simulink model "FDM_Degradation_oglm"  (R2020b)
settings: Solver=ode23tb  StartTime=0.0  StopTime=t_final  MaxStep=0.1  RelTol=1e-3
values from neighbouring files (symbols this model uses):
  initial_50_n = [0.015535 0.015535 0.015535 0.015535 0.015535 0.015535 0.015535 0.015535 0.015535 0.015535 0.015535 0.015535 ... (49 elements, 1x49)]    [LM_0.mat]    (also in RUn_Model_FDM.m = repmat(C_avg_n, 1, 49))
settings Model: Creator=moonjihoon  LastModifiedBy=moonjihoon

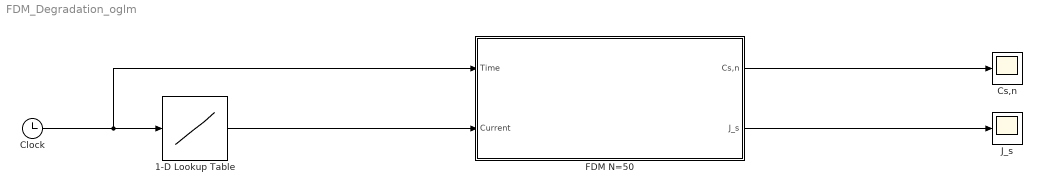
== system FDM_Degradation_oglm ==
  1-D Lookup Table : Lookup_n-D  NumberOfTableDimensions=1  BreakpointsForDimension1=t  Table=u  InternalRulePriority=Speed  RndMeth=Simplest  InputSameDT=on
  Clock : Clock
  Cs,n : Scope
  "FDM N=50 " : Subsystem
  J_s : Scope
  wires:
  1-D Lookup Table/1 -> "FDM N=50 "/2(Current)
  Clock/1 -> 1-D Lookup Table/1, "FDM N=50 "/1(Time)
  "FDM N=50 "/2(J_s) -> J_s/1
  "FDM N=50 "/1(Cs,n) -> Cs,n/1

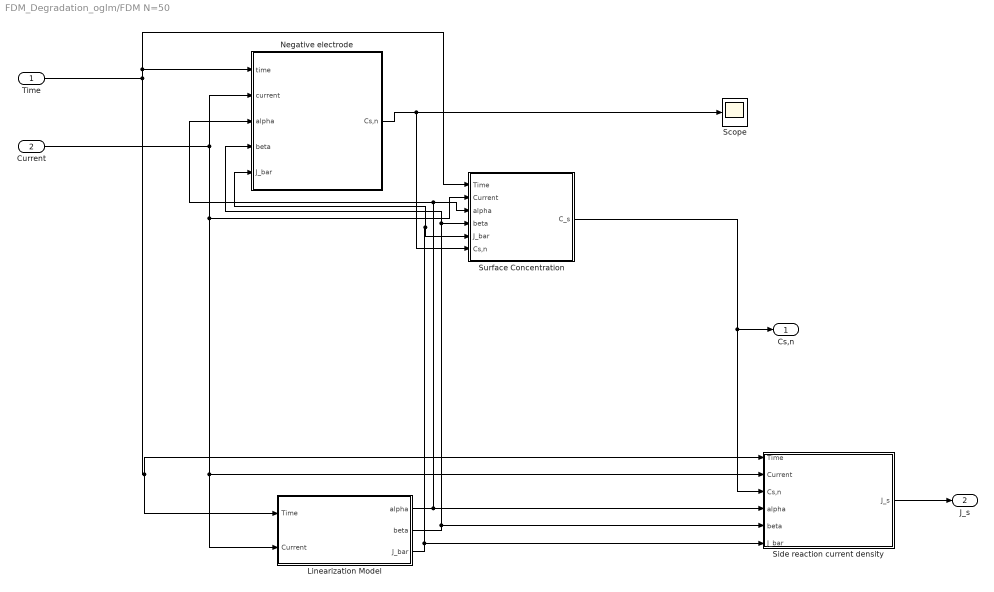
== system FDM_Degradation_oglm/FDM N=50  ==
  Time : Inport
  Current : Inport  Port=2
  Linearization Model : Subsystem
  Negative electrode : Subsystem
  Scope : Scope
  Side reaction current density : Subsystem
  Surface Concentration : Subsystem
  Cs,n : Outport
  J_s : Outport  Port=2
  wires:
  Negative electrode/1(Cs,n) -> Scope/1, Surface Concentration/6(Cs,n)
  Linearization Model/2(beta) -> Side reaction current density/5(beta), Negative electrode/4(beta), Surface Concentration/4(beta)
  Side reaction current density/1(J_s) -> J_s/1
  Linearization Model/1(alpha) -> Side reaction current density/4(alpha), Negative electrode/3(alpha), Surface Concentration/3(alpha)
  Time/1 -> Surface Concentration/1(Time), Negative electrode/1(time), Linearization Model/1(Time), Side reaction current density/1(Time)
  Surface Concentration/1(C_s) -> Side reaction current density/3(Cs,n), Cs,n/1
  Linearization Model/3(J_bar) -> Side reaction current density/6(J_bar), Negative electrode/5(J_bar), Surface Concentration/5(J_bar)
  Current/1 -> Surface Concentration/2(Current), Linearization Model/2(Current), Side reaction current density/2(Current), Negative electrode/2(current)

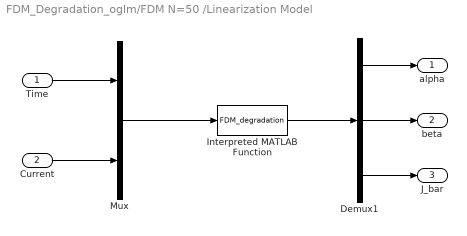
== system FDM_Degradation_oglm/FDM N=50 /Linearization Model ==
  Time : Inport
  Current : Inport  Port=2
  Demux1 : Demux  Outputs=3
  Interpreted MATLAB Function : MATLABFcn  MATLABFcn=FDM_degradation
  Mux : Mux  Inputs=2
  alpha : Outport
  beta : Outport  Port=2
  J_bar : Outport  Port=3
  wires:
  Demux1/1 -> alpha/1
  Demux1/3 -> J_bar/1
  Current/1 -> Mux/2
  Time/1 -> Mux/1
  Interpreted MATLAB Function/1 -> Demux1/1
  Demux1/2 -> beta/1
  Mux/1 -> Interpreted MATLAB Function/1

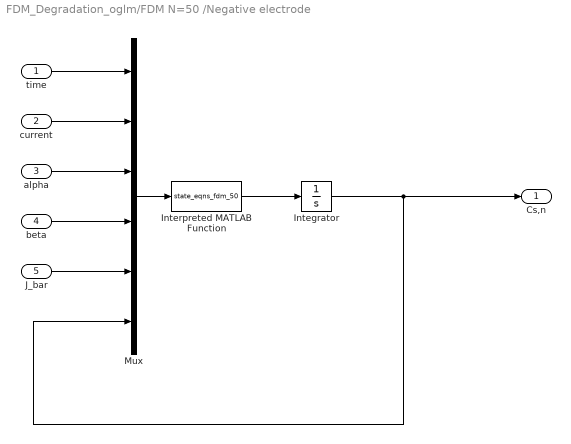
== system FDM_Degradation_oglm/FDM N=50 /Negative electrode ==
  time : Inport
  current : Inport  Port=2
  alpha : Inport  Port=3
  beta : Inport  Port=4
  J_bar : Inport  Port=5
  Integrator : Integrator  InitialCondition=initial_50_n
  Interpreted MATLAB Function : MATLABFcn  MATLABFcn=state_eqns_fdm_50
  Mux : Mux  Inputs=6
  Cs,n : Outport
  wires:
  Interpreted MATLAB Function/1 -> Integrator/1
  time/1 -> Mux/1
  current/1 -> Mux/2
  Mux/1 -> Interpreted MATLAB Function/1
  Integrator/1 -> Mux/6, Cs,n/1
  J_bar/1 -> Mux/5
  beta/1 -> Mux/4
  alpha/1 -> Mux/3

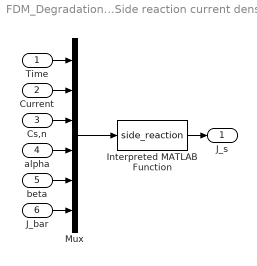
== system FDM_Degradation_oglm/FDM N=50 /Side reaction current density ==
  Time : Inport
  Current : Inport  Port=2
  Cs,n : Inport  Port=3
  alpha : Inport  Port=4
  beta : Inport  Port=5
  J_bar : Inport  Port=6
  Interpreted MATLAB Function : MATLABFcn  MATLABFcn=side_reaction
  Mux : Mux  Inputs=6
  J_s : Outport
  wires:
  Interpreted MATLAB Function/1 -> J_s/1
  Time/1 -> Mux/1
  Current/1 -> Mux/2
  Mux/1 -> Interpreted MATLAB Function/1
  J_bar/1 -> Mux/6
  beta/1 -> Mux/5
  alpha/1 -> Mux/4
  Cs,n/1 -> Mux/3

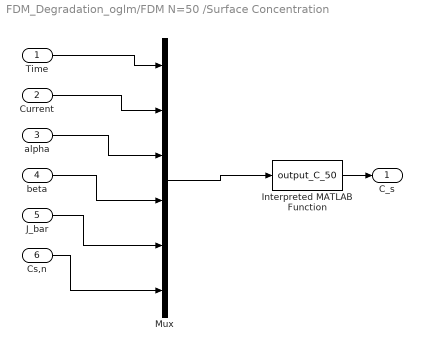
== system FDM_Degradation_oglm/FDM N=50 /Surface Concentration ==
  Time : Inport
  Current : Inport  Port=2
  alpha : Inport  Port=3
  beta : Inport  Port=4
  J_bar : Inport  Port=5
  Cs,n : Inport  Port=6
  Interpreted MATLAB Function : MATLABFcn  MATLABFcn=output_C_50
  Mux : Mux  Inputs=6
  C_s : Outport
  wires:
  Interpreted MATLAB Function/1 -> C_s/1
  beta/1 -> Mux/4
  J_bar/1 -> Mux/5
  alpha/1 -> Mux/3
  Cs,n/1 -> Mux/6
  Current/1 -> Mux/2
  Mux/1 -> Interpreted MATLAB Function/1
  Time/1 -> Mux/1
